simulink model "Poject_PilotInLoop_Beech_99_Nonlinear_Simulation_Turn_f"  (R2018b)
settings: Solver=ode45  StartTime=0.0  StopTime=3000  RelTol=1e-3
InitFcn:
  | Initial_Data_Coordinate_Turn
StopFcn:
  | Plots_Coordinate_Turn
undefined symbols (not defined in the file or in its folder): b, c, CD0, CDalpha, CDalphadot, CDdelE, CDiH, CDq, CDu, CL0, CLalpha, CLalphadot, Clbeta, Clbetadot, CldelA, CLdelE, CldelR, CLiH, Clp, CLq, Clr, ClT, CLu, Cm0, Cmalpha, Cmalphadot, CmdelE, cmiH, Cmq, CmT1, CmTalpha, CmTu, Cmu, Cnbeta, Cnbetadot, CndelA, CndelR, Cnp, Cnr, CnTbeta, CTxu, CTy, CTz, Cybeta, Cybetadot, CydelA, CydelR, Cyp, Cyr, g, iH, Ixx, Ixz, Iyy, Izz, Kp, mass, Ro, S, T1 ... (+4)
libraries: simulink x1
(part 2 of 2)

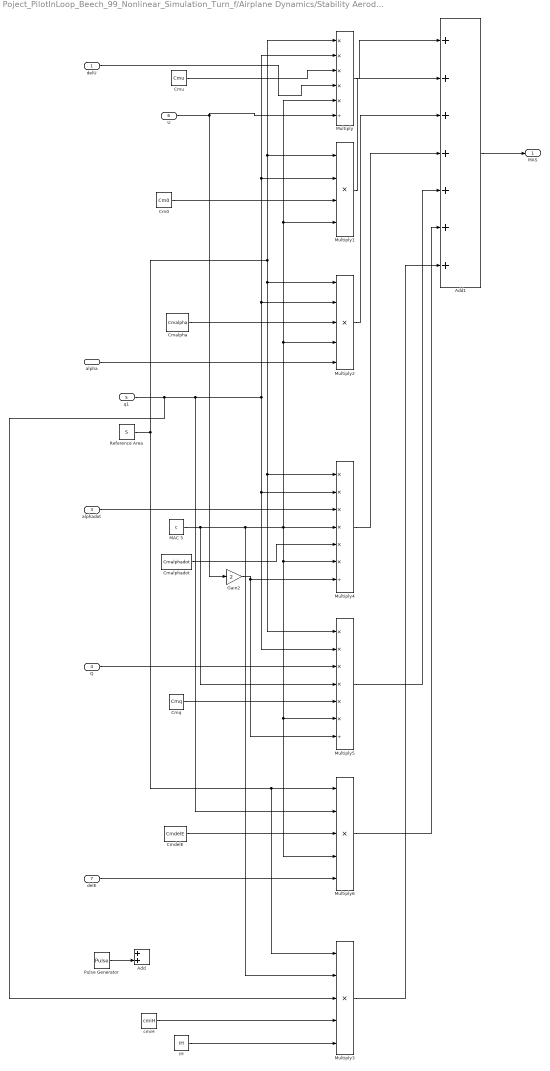
== system Poject_PilotInLoop_Beech_99_Nonlinear_Simulation_Turn_f/Airplane Dynamics/Stability Aerodunamic Forces and Moments (FAxS,FAyS,FAzS,LAS,MAS,NAS)/MASBlock1 ==
  delU : Inport
  alpha : Inport  Port=2
  alphadot : Inport  Port=3
  Q : Inport  Port=4
  q1 : Inport  Port=5
  U : Inport  Port=6
  delE : Inport  Port=7
  Add : Sum
  Add1 : Sum  Inputs=+++++++
  Cm0 : Constant  Value=Cm0
  Cmalpha : Constant  Value=Cmalpha
  Cmalphadot : Constant  Value=Cmalphadot
  CmdelE : Constant  Value=CmdelE
  Cmq : Constant  Value=Cmq
  Cmu : Constant  Value=Cmu
  Gain2 : Gain  Gain=2
  MAC 5 : Constant  Value=c
  Multiply : Product  Inputs=*****/
  Multiply1 : Product  Inputs=****
  Multiply2 : Product  Inputs=*****
  Multiply3 : Product  Inputs=*****
  Multiply4 : Product  Inputs=******/
  Multiply5 : Product  Inputs=******/
  Multiply6 : Product  Inputs=*****
  Pulse Generator : DiscretePulseGenerator  PulseType=Time based  Amplitude=0.035  Period=2000  PulseWidth=0.05
  "Reference Area " : Constant  Value=S
  cmiH : Constant  Value=cmiH
  iH : Constant  Value=iH
  MAS : Outport
  wires:
  U/1 -> Multiply/6, Gain2/1
  q1/1 -> Multiply3/3, Multiply6/2, Multiply/2, Multiply1/2, Multiply2/2, Multiply5/2, Multiply4/2
  delU/1 -> Multiply/4
  "Reference Area "/1 -> Multiply6/1, Multiply3/1, Multiply5/1, Multiply4/1, Multiply2/1, Multiply/1, Multiply1/1
  alphadot/1 -> Multiply4/3
  Q/1 -> Multiply5/3
  MAC 5/1 -> Multiply5/4, Multiply3/2, Multiply6/4, Multiply5/6, Multiply4/6, Multiply/5, Multiply1/4, Multiply2/4, Multiply4/4
  alpha/1 -> Multiply2/5
  Add1/1 -> MAS/1
  Multiply/1 -> Add1/1
  Cmq/1 -> Multiply5/5
  Cmalphadot/1 -> Multiply4/5
  Multiply5/1 -> Add1/5
  Gain2/1 -> Multiply5/7, Multiply4/7
  Multiply1/1 -> Add1/2
  Multiply2/1 -> Add1/3
  Cmu/1 -> Multiply/3
  Cmalpha/1 -> Multiply2/3
  CmdelE/1 -> Multiply6/3
  Multiply6/1 -> Add1/6
  Multiply4/1 -> Add1/4
  Cm0/1 -> Multiply1/3
  cmiH/1 -> Multiply3/4
  iH/1 -> Multiply3/5
  Multiply3/1 -> Add1/7
  delE/1 -> Multiply6/5
  Pulse Generator/1 -> Add/2

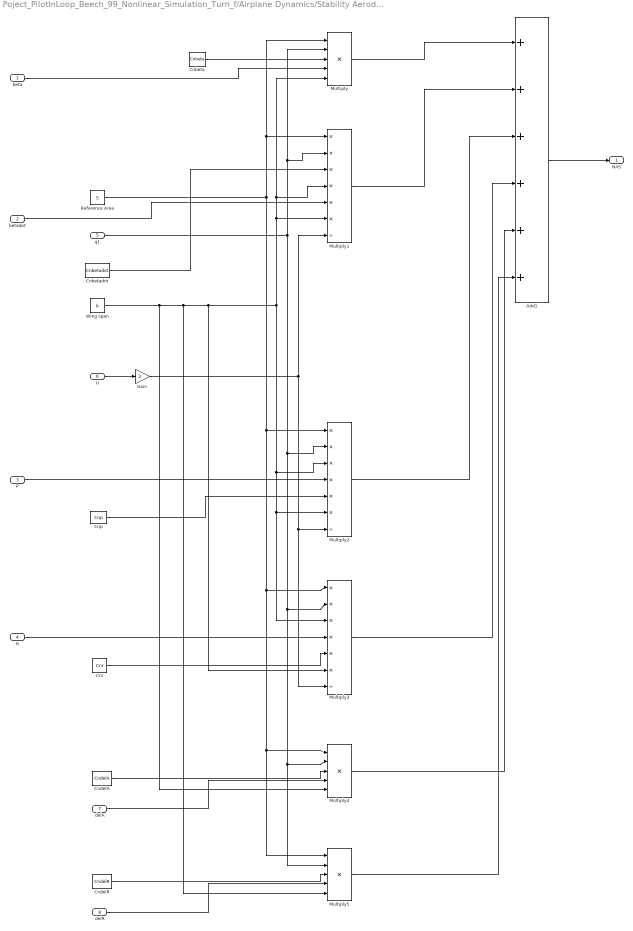
== system Poject_PilotInLoop_Beech_99_Nonlinear_Simulation_Turn_f/Airplane Dynamics/Stability Aerodunamic Forces and Moments (FAxS,FAyS,FAzS,LAS,MAS,NAS)/NASBlock ==
  beta : Inport
  betadot : Inport  Port=2
  P : Inport  Port=3
  R : Inport  Port=4
  q1 : Inport  Port=5
  U : Inport  Port=6
  delA : Inport  Port=7
  delR : Inport  Port=8
  Add1 : Sum  Inputs=++++++
  Cnbeta : Constant  Value=Cnbeta
  Cnbetadot : Constant  Value=Cnbetadot
  CndelA : Constant  Value=CndelA
  CndelR : Constant  Value=CndelR
  Cnp : Constant  Value=Cnp
  Cnr : Constant  Value=Cnr
  Gain : Gain  Gain=2
  Multiply : Product  Inputs=*****
  Multiply1 : Product  Inputs=******/
  Multiply2 : Product  Inputs=******/
  Multiply3 : Product  Inputs=******/
  Multiply4 : Product  Inputs=*****
  Multiply5 : Product  Inputs=*****
  Reference Area : Constant  Value=S
  Wing span : Constant  Value=b
  NAS : Outport
  wires:
  U/1 -> Gain/1
  Multiply3/1 -> Add1/4
  Cnbeta/1 -> Multiply/3
  Multiply/1 -> Add1/1
  beta/1 -> Multiply/4
  Multiply2/1 -> Add1/3
  Cnr/1 -> Multiply3/5
  R/1 -> Multiply3/4
  Multiply4/1 -> Add1/5
  P/1 -> Multiply2/4
  delR/1 -> Multiply5/4
  Multiply1/1 -> Add1/2
  q1/1 -> Multiply1/2, Multiply/2, Multiply2/2, Multiply3/2, Multiply4/2, Multiply5/2
  Gain/1 -> Multiply2/7, Multiply3/7, Multiply1/7
  CndelA/1 -> Multiply4/3
  betadot/1 -> Multiply1/5
  Wing span/1 -> Multiply1/6, Multiply/5, Multiply1/4, Multiply2/3, Multiply3/3, Multiply2/6, Multiply3/6, Multiply5/5, Multiply4/5
  Add1/1 -> NAS/1
  Reference Area/1 -> Multiply1/1, Multiply/1, Multiply2/1, Multiply3/1, Multiply4/1, Multiply5/1
  Cnp/1 -> Multiply2/5
  delA/1 -> Multiply4/4
  Multiply5/1 -> Add1/6
  Cnbetadot/1 -> Multiply1/3
  CndelR/1 -> Multiply5/3

== system Poject_PilotInLoop_Beech_99_Nonlinear_Simulation_Turn_f/Airplane Dynamics/Thrust Forces and Moments (FTx,FTy,FTz,LT,MT,NT)/FTxBlock ==
  delU : Inport
  q1 : Inport  Port=2
  U : Inport  Port=3
  Add : Sum
  Add1 : Sum
  CTxu : Constant  Value=CTxu
  Multiply : Product  Inputs=****/
  Multiply1 : Product
  Pulse Generator : DiscretePulseGenerator  PulseType=Time based  Amplitude=0.05  Period=2000  PulseWidth=0.05
  Refernce Area : Constant  Value=S
  Scope : Scope
  T_trim : Constant  Value=T1
  FTx : Outport
  wires:
  delU/1 -> Multiply/4
  Multiply/1 -> Add1/1
  U/1 -> Multiply/5
  CTxu/1 -> Multiply/3
  Refernce Area/1 -> Multiply/1
  q1/1 -> Multiply/2
  T_trim/1 -> Add1/2
  Pulse Generator/1 -> Scope/1, Multiply1/2
  Multiply1/1 -> Add/2
  Add1/1 -> FTx/1

== system Poject_PilotInLoop_Beech_99_Nonlinear_Simulation_Turn_f/Airplane Dynamics/Thrust Forces and Moments (FTx,FTy,FTz,LT,MT,NT)/FTyBlock ==
  q1 : Inport
  CTy : Constant  Value=CTy
  Multiply : Product  Inputs=***
  Refernce Area : Constant  Value=S
  FTy : Outport
  wires:
  Multiply/1 -> FTy/1
  q1/1 -> Multiply/2
  Refernce Area/1 -> Multiply/1
  CTy/1 -> Multiply/3

== system Poject_PilotInLoop_Beech_99_Nonlinear_Simulation_Turn_f/Airplane Dynamics/Thrust Forces and Moments (FTx,FTy,FTz,LT,MT,NT)/FTzBlock ==
  q1 : Inport
  CTz : Constant  Value=CTz
  Multiply : Product  Inputs=***
  Refernce Area : Constant  Value=S
  FTz : Outport
  wires:
  CTz/1 -> Multiply/3
  Refernce Area/1 -> Multiply/1
  q1/1 -> Multiply/2
  Multiply/1 -> FTz/1

== system Poject_PilotInLoop_Beech_99_Nonlinear_Simulation_Turn_f/Airplane Dynamics/Thrust Forces and Moments (FTx,FTy,FTz,LT,MT,NT)/LTBlock ==
  q1 : Inport
  ClT : Constant  Value=ClT
  Multiply : Product  Inputs=****
  Refernce Area : Constant  Value=S
  Wing span : Constant  Value=b
  LT : Outport
  wires:
  ClT/1 -> Multiply/3
  Refernce Area/1 -> Multiply/1
  q1/1 -> Multiply/2
  Multiply/1 -> LT/1
  Wing span/1 -> Multiply/4

== system Poject_PilotInLoop_Beech_99_Nonlinear_Simulation_Turn_f/Airplane Dynamics/Thrust Forces and Moments (FTx,FTy,FTz,LT,MT,NT)/MTBlock ==
  delU : Inport
  alpha : Inport  Port=2
  q1 : Inport  Port=3
  U : Inport  Port=4
  Add1 : Sum  Inputs=+++
  CmT1 : Constant  Value=CmT1
  CmTalpha : Constant  Value=CmTalpha
  CmTu : Constant  Value=CmTu
  Gain : Gain  Gain=2
  MAC : Constant  Value=c
  Multiply : Product  Inputs=*****/
  Multiply1 : Product  Inputs=*****/
  Multiply2 : Product  Inputs=*****
  Refernce Area : Constant  Value=S
  MT : Outport
  wires:
  Gain/1 -> Multiply1/3
  Add1/1 -> MT/1
  q1/1 -> Multiply2/2, Multiply1/2, Multiply/2
  Multiply1/1 -> Add1/2
  Refernce Area/1 -> Multiply2/1, Multiply1/1, Multiply/1
  CmTu/1 -> Multiply/3
  CmT1/1 -> Gain/1
  U/1 -> Multiply1/6, Multiply/6
  Multiply/1 -> Add1/1
  delU/1 -> Multiply1/4, Multiply/4
  Multiply2/1 -> Add1/3
  MAC/1 -> Multiply2/3, Multiply1/5, Multiply/5
  alpha/1 -> Multiply2/4
  CmTalpha/1 -> Multiply2/5

== system Poject_PilotInLoop_Beech_99_Nonlinear_Simulation_Turn_f/Airplane Dynamics/Thrust Forces and Moments (FTx,FTy,FTz,LT,MT,NT)/NTBlock ==
  beta : Inport
  q1 : Inport  Port=2
  CnTbeta : Constant  Value=CnTbeta
  Multiply : Product  Inputs=*****
  Refernce Area : Constant  Value=S
  Wing span : Constant  Value=b
  NT : Outport
  wires:
  Multiply/1 -> NT/1
  q1/1 -> Multiply/2
  Refernce Area/1 -> Multiply/1
  CnTbeta/1 -> Multiply/3
  Wing span/1 -> Multiply/5
  beta/1 -> Multiply/4
